simulink model "czwartasymulacja"  (R2024a)
settings: Solver=VariableStepAuto  StartTime=0.0  StopTime=150000  RelTol=1e-3
libraries: fl_lib x3, nesl_utility x3, BatteryCurrentManagement x1, batt_lib x1, BatteryEstimators x1
settings Model: Creator=jakub  LastModifiedBy=jakub

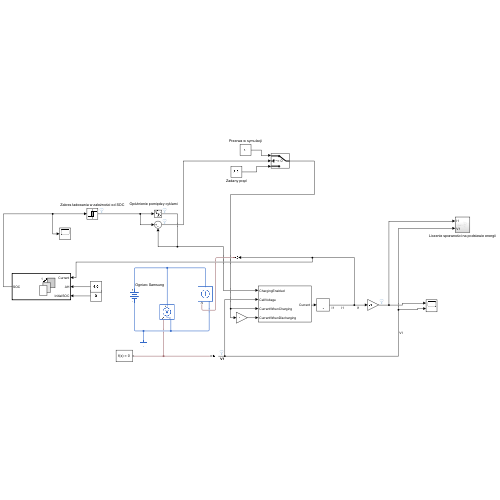
[thumbnail: Simulink's stored preview of the top-level diagram]
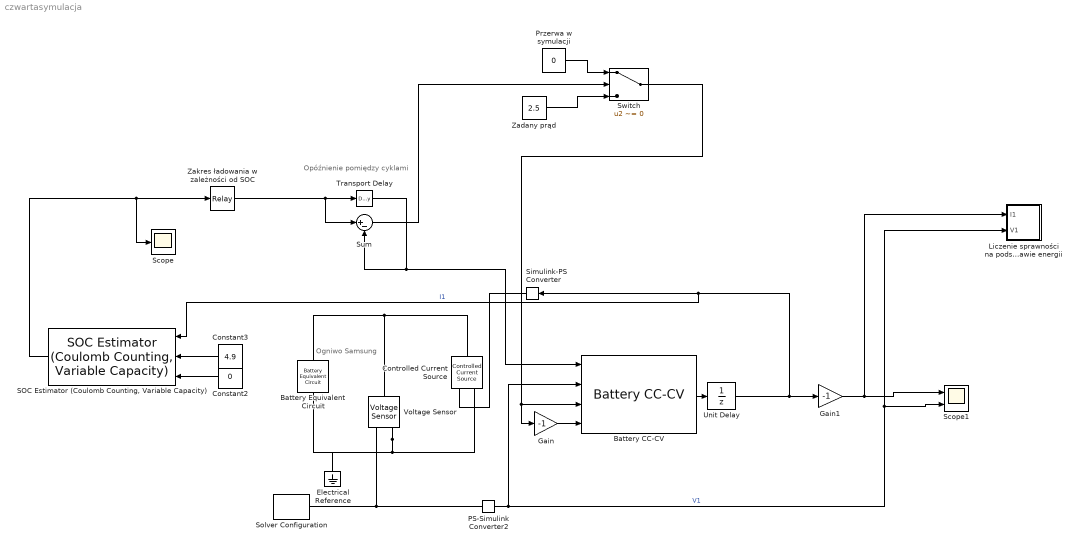
== system czwartasymulacja ==
  note: Ogniwo Samsung
  note: Opóźnienie pomiędzy cyklami
  Battery CC-CV : BatteryCurrentManagement/Battery CC-CV  MaxCellVoltage=4.28  Kp=1  Ki=5  Kaw=1  Kt=1  Ts=1
      settings: LibrarySourceBlock=batt_sl_lib/Current Management/Battery CC-CV
  Battery Equivalent Circuit : batt_lib/Cells/Battery Equivalent Circuit  BatteryCapacity=4900 mAh  ThermalModel=simscape.battery.enum.cells.BatteryThermalModel.ConstantTemperature  ExtrapolationMethod=simscape.enum.extrapolation.nearest  EnableFaultExotherm=false  TriggerTemperature=350 K  SOCBreakpoints=[0.01, 0.04, 0.06, 0.09, 0.11, 0.14, 0.16, 0.19, 0.21, 0.24, 0.26, 0.29, 0.31, 0.34, 0.36, 0.39, 0.41, 0.44, 0.46, 0.49, 0.51, 0.54, 0.56, 0.59, 0.61, 0.64, 0.66, 0.69, 0.71, 0.74, 0.76, 0.79, 0.81, 0.84, 0.86, 0.89]  TemperatureBreakpoints=[278, 293, 313] K  OpenCircuitVoltage=[3.5057, 3.566, 3.6337, 3.7127, 3.9259, 4.0777, 4.1928] V  OpenCircuitVoltageThermal=|  VoltageRange=[0, inf] V  HysteresisModel=simscape.battery.enum.cells.HysteresisModel.none  MaximumHysteresisVoltage=[0, 0, 0, 0, 0, 0, 0] V  InstantaneousHysteresisVoltage=[0, 0, 0, 0, 0, 0, 0] V  HysteresisRate=0.1  MaximumHysteresisVoltageThermal=[0, 0, 0; 0, 0, 0; 0, 0, 0; 0, 0, 0; 0, 0, 0; 0, 0, 0; 0, 0, 0] V  InstantaneousHysteresisVoltageThermal=[0, 0, 0; 0, 0, 0; 0, 0, 0; 0, 0, 0; 0, 0, 0; 0, 0, 0; 0, 0, 0] V  HysteresisRateThermal=0.1  ResistanceSOCBreakpoints=[.01, .1, .25, .5, .75, .9, 1]  ResistanceTemperatureBreakpoints=[278, 293, 313] K  CurrentDirectionality=simscape.battery.enum.cells.BatteryEnable.Disabled  R0=[.0085, .0085, .0087, .0082, .0083, .0085, .0085] Ohm  R0Thermal=|  DischargeR0=[.0085, .0085, .0087, .0082, .0083, .0085, .0085] Ohm  ChargeR0=[.0085, .0085, .0087, .0082, .0083, .0085, .0085] Ohm  ChargeR0Thermal=|  DischargeR0Thermal=|  SelfDischargeResistor=simscape.battery.enum.cells.BatteryEnable.Disabled  SelfDischargeR=7e3 Ohm  SelfDischargeRThermal=[8000, 7000, 6000] Ohm  RCPairs=simscape.battery.enum.cells.RCPairs.noDynamics  R1=[.0029, .0024, .0026, .0016, .0023, .0018, .0017] Ohm  Tau1=[36, 45, 105, 29, 77, 33, 39] s  R2=[.0029, .0024, .0026, .0016, .0023, .0018, .0017] Ohm  Tau2=[36, 45, 105, 29, 77, 33, 39] s  R3=[.0029, .0024, .0026, .0016, .0023, .0018, .0017] Ohm  Tau3=[36, 45, 105, 29, 77, 33, 39] s  DischargeR1=[.0029, .0024, .0026, .0016, .0023, .0018, .0017] Ohm  DischargeTau1=[36, 45, 105, 29, 77, 33, 39] s  ChargeR1=[.0029, .0024, .0026, .0016, .0023, .0018, .0017] Ohm  ChargeTau1=[36, 45, 105, 29, 77, 33, 39] s  DischargeR2=[.0029, .0024, .0026, .0016, .0023, .0018, .0017] Ohm  DischargeTau2=[36, 45, 105, 29, 77, 33, 39] s  ChargeR2=[.0029, .0024, .0026, .0016, .0023, .0018, .0017] Ohm  ChargeTau2=[36, 45, 105, 29, 77, 33, 39] s  DischargeR3=[.0029, .0024, .0026, .0016, .0023, .0018, .0017] Ohm  DischargeTau3=[36, 45, 105, 29, 77, 33, 39] s  ChargeR3=[.0029, .0024, .0026, .0016, .0023, .0018, .0017] Ohm  ChargeTau3=[36, 45, 105, 29, 77, 33, 39] s  R1Thermal=[.0109, .0029, .0013; .0069, .0024, .0012; .0047, .0026, .0013; .0034, .0016, .001; .0033, .0023, .0014; .0033, .0018, .0011; .0028, .0017, .0011] Ohm  Tau1Thermal=[20, 36, 39; 31, 45, 39; 109, 105, 61; 36, 29, 26; 59, 77, 67; 40, 33, 29; 25, 39, 33] s  R2Thermal=[.0109, .0029, .0013; .0069, .0024, .0012; .0047, .0026, .0013; .0034, .0016, .001; .0033, .0023, .0014; .0033, .0018, .0011; .0028, .0017, .0011] Ohm  Tau2Thermal=[20, 36, 39; 31, 45, 39; 109, 105, 61; 36, 29, 26; 59, 77, 67; 40, 33, 29; 25, 39, 33] s  R3Thermal=[.0109, .0029, .0013; .0069, .0024, .0012; .0047, .0026, .0013; .0034, .0016, .001; .0033, .0023, .0014; .0033, .0018, .0011; .0028, .0017, .0011] Ohm  Tau3Thermal=[20, 36, 39; 31, 45, 39; 109, 105, 61; 36, 29, 26; 59, 77, 67; 40, 33, 29; 25, 39, 33] s  DischargeR1Thermal=[.0109, .0029, .0013; .0069, .0024, .0012; .0047, .0026, .0013; .0034, .0016, .001; .0033, .0023, .0014; .0033, .0018, .0011; .0028, .0017, .0011] Ohm  DischargeTau1Thermal=[20, 36, 39; 31, 45, 39; 109, 105, 61; 36, 29, 26; 59, 77, 67; 40, 33, 29; 25, 39, 33] s  ChargeR1Thermal=[.0109, .0029, .0013; .0069, .0024, .0012; .0047, .0026, .0013; .0034, .0016, .001; .0033, .0023, .0014; .0033, .0018, .0011; .0028, .0017, .0011] Ohm  ChargeTau1Thermal=[20, 36, 39; 31, 45, 39; 109, 105, 61; 36, 29, 26; 59, 77, 67; 40, 33, 29; 25, 39, 33] s  DischargeR2Thermal=[.0109, .0029, .0013; .0069, .0024, .0012; .0047, .0026, .0013; .0034, .0016, .001; .0033, .0023, .0014; .0033, .0018, .0011; .0028, .0017, .0011] Ohm  DischargeTau2Thermal=[20, 36, 39; 31, 45, 39; 109, 105, 61; 36, 29, 26; 59, 77, 67; 40, 33, 29; 25, 39, 33] s  ChargeR2Thermal=[.0109, .0029, .0013; .0069, .0024, .0012; .0047, .0026, .0013; .0034, .0016, .001; .0033, .0023, .0014; .0033, .0018, .0011; .0028, .0017, .0011] Ohm  ChargeTau2Thermal=[20, 36, 39; 31, 45, 39; 109, 105, 61; 36, 29, 26; 59, 77, 67; 40, 33, 29; 25, 39, 33] s  DischargeR3Thermal=[.0109, .0029, .0013; .0069, .0024, .0012; .0047, .0026, .0013; .0034, .0016, .001; .0033, .0023, .0014; .0033, .0018, .0011; .0028, .0017, .0011] Ohm  DischargeTau3Thermal=[20, 36, 39; 31, 45, 39; 109, 105, 61; 36, 29, 26; 59, 77, 67; 40, 33, 29; 25, 39, 33] s  ChargeR3Thermal=[.0109, .0029, .0013; .0069, .0024, .0012; .0047, .0026, .0013; .0034, .0016, .001; .0033, .0023, .0014; .0033, .0018, .0011; .0028, .0017, .0011] Ohm  ChargeTau3Thermal=[20, 36, 39; 31, 45, 39; 109, 105, 61; 36, 29, 26; 59, 77, 67; 40, 33, 29; 25, 39, 33] s  CyclingAgingMethod=simscape.battery.enum.cells.CyclingAgingMethod.disabled  NumDisCycles=100  OCVChange=0  R0Change=0  CapacityChange=0  SelfDischargeRChange=0  R1Change=0  R2Change=0  R3Change=0  NumDisCyclesBreakpoints=[0, 100, 200, 300]  AgingTemperatureBreakpoints=[298.15, 323.15] K  OCVChangeVec=[0, 0, 0, 0]  R0ChangeVec=[0, 0, 0, 0]  CapacityChangeVec=[0, 0, 0, 0]  SelfDischargeRChangeVec=[0, 0, 0, 0]  R1ChangeVec=[0, 0, 0, 0]  R2ChangeVec=[0, 0, 0, 0]  R3ChangeVec=[0, 0, 0, 0]  OCVChangeThermal=[0, 0; 0, 0; 0, 0; 0, 0]  R0ChangeThermal=[0, 0; 0, 0; 0, 0; 0, 0]  CapacityChangeThermal=[0, 0; 0, 0; 0, 0; 0, 0]  SelfDischargeRChangeThermal=[0, 0; 0, 0; 0, 0; 0, 0]  R1ChangeThermal=[0, 0; 0, 0; 0, 0; 0, 0]  R2ChangeThermal=[0, 0; 0, 0; 0, 0; 0, 0]  R3ChangeThermal=[0, 0; 0, 0; 0, 0; 0, 0]  CalendarAgeResistance=simscape.battery.enum.cells.BatteryEnable.Disabled  CalendarAgeCapacity=simscape.battery.enum.cells.BatteryEnable.Disabled  CalendarAgingMethod=simscape.battery.enum.cells.CalendarAgingMethod.equation  StorageVariable=simscape.battery.enum.cells.StorageVariable.OCV  OCVDuringStorage=0.9  SOCDuringStorage=0.6  StorageTimeIntervals=[0] d  StorageTemperatures=[273] K  ResistanceScalingOCV=2.2134e6  ResistanceScalingOCVOffset=1.632e6  ResistanceExponentialIncrease=0.515833569 V  ResistanceTimeExponent=0.75  ResistanceAgeTemperatureBreakpoints=[273.15, 298.15, 323.15] K  ResistanceAgeTimeBreakpoints=[0, 90, 180, 270] d  PercentResistanceChange=[0, 0, 0]  ResistanceTimeBreakpoints=100 d  PercentResistanceChangeThermal=[0, 0, 0; 0, 0, 0; 0, 0, 0; 0, 0, 0]  CapacityScalingOCV=1.5097e07  CapacityScalingOCVOffset=8.3625e06  CapacityExponentialIncrease=0.6011 V  CapacityTimeExponent=0.75  CapacityAgeTemperatureBreakpoints=[273.15, 298.15, 323.15] K  CapacityAgeTimeBreakpoints=[0, 90, 180, 270] d  PercentCapacityChange=[0, 0, 0]  CapacityTimeBreakpoints=100 d  PercentCapacityChangeThermal=[0, 0, 0; 0, 0, 0; 0, 0, 0; 0, 0, 0]  SimulationTemperature=298.15 K  BatteryThermalMass=100 J/K  ReversibleHeatModel=simscape.battery.enum.cells.ReversibleHeatModel.Disabled  EntropicCoefficient=[0, 0, 0, 0, 0, 0, 0] mV/K  AddedResistance=1e5 Ohm  ShortedResistance=1e-6 Ohm  ExothermModel=simscape.battery.enum.cells.ExothermModel.analytical  TabulateWithSOC=false  SOCvecExotherm=[0, .5, 1]  CurrInterruptTempSOC=[420, 420, 420] K  TotalHeatOfReactionSOC=[23000, 23000, 23000] J  CurrentInterruptTemperature=420 K  TotalHeatOfReaction=23e3 J  ExothermOnsetTemperature=350 K  ExothermOnsetTempSOC=[350, 350, 350] K  OnsetTempRate=0.02 K/min  ActivationEnergy=160e3 J/mol  ActivationEnergySOC=[160000, 160000, 160000] J/mol  ReactionOrder=1  ReactionOrderSOC=[1, 1, 1]  TemperaturesFromARC=[323, 373, 423, 438, 463, 483, 513, 543, 545, 547, 549, 551, 553, 573, 623, 773, 923, 943, 1003, 1063, 1113, 1123, 1133, 1153, 1173] K  TemperatureRatesFromARC=[.0001, .001, .025, .2, .4, .6, 1.1, 1.3, 1.9, 3, 5, 11.6, 183.3, 191.6, 200, 208.3, 200, 175, 8.33, 1.33, .33, .2, .13, .0017, .00017] K/s  TempRateVecARCSOC=repmat([.0001, .001, .025, .2, .4, .6, 1.1, 1.3, 1.9, 3, 5, 11.6, 183.3, 191.6, 200, 208.3, 200, 175, 8.33, 1.33, .33, .2, .13, .0017, .00017]', 1, 3) K/s  PercentThermalMassVented=40  PercentThermalMassVentedSOC=[40, 40, 40]  EnableFaultAddRes=false  EnableFaultShort=false  faultTriggerType=simscape.fault.triggertype.external  stateOfCharge_specify=on  stateOfCharge_priority=High  stateOfCharge=0  stateOfCharge_nominal_specify=off  stateOfCharge_nominal_value=1  stateOfCharge_nominal_unit=1  numCycles_specify=off  numCycles_priority=High  numCycles=0.1  numCycles_nominal_specify=off  numCycles_nominal_value=1  numCycles_nominal_unit=1  batteryVoltage_specify=off  batteryVoltage_priority=None  batteryVoltage=0 V  batteryVoltage_nominal_specify=off  batteryVoltage_nominal_value=1  batteryVoltage_nominal_unit=V  batteryCurrent_specify=off  batteryCurrent_priority=None  batteryCurrent=0 A  batteryCurrent_nominal_specify=off  batteryCurrent_nominal_value=1  batteryCurrent_nominal_unit=A  batteryTemperature_specify=off  batteryTemperature_priority=High  batteryTemperature=298.15 K  batteryTemperature_nominal_specify=off  batteryTemperature_nominal_value=1  batteryTemperature_nominal_unit=K  hysteresisState_specify=off  hysteresisState_priority=High  hysteresisState=0  hysteresisState_nominal_specify=off  hysteresisState_nominal_value=1  hysteresisState_nominal_unit=1  isExothermFaulted_specify=off  isExothermFaulted_priority=None  isExothermFaulted=0  isExothermFaulted_nominal_specify=off  isExothermFaulted_nominal_value=1  isExothermFaulted_nominal_unit=1  isCurrentInterruptionTempExceeded_specify=off  isCurrentInterruptionTempExceeded_priority=None  isCurrentInterruptionTempExceeded=0  isCurrentInterruptionTempExceeded_nominal_specify=off  isCurrentInterruptionTempExceeded_nominal_value=1  isCurrentInterruptionTempExceeded_nominal_unit=1  reactionHeatRate_specify=off  reactionHeatRate_priority=None  reactionHeatRate=0 W  reactionHeatRate_nominal_specify=off  reactionHeatRate_nominal_value=1  reactionHeatRate_nominal_unit=W  reactionExtent_specify=off  reactionExtent_priority=None  reactionExtent=0  reactionExtent_nominal_specify=off  reactionExtent_nominal_value=1  reactionExtent_nominal_unit=1
      OpenCircuitVoltageThermal=|
      | [
      |        2.60, 2.58, 2.55;
      |        2.78, 2.76, 2.73;
      |        2.96, 2.94, 2.91;
      |        3.14, 3.11, 3.09;
      |        3.27, 3.24, 3.22;
      |        3.31, 3.28, 3.26;
      |        3.35, 3.33, 3.30;
      |        3.39, 3.37, 3.34;
      |        3.42, 3.40, 3.37;
      |        3.44, 3.42, 3.39;
      |        3.46, 3.44, 3.41;
      |        3.49, 3.47, 3.44;
      |        3.51, 3.49, 3.46;
      |        3.54, 3.52, 3.48;
      |        3.56, 3.54, 3.51;
      |        3.58, 3.56, 3.53;
      |        3.61, 3.59, 3.56;
      |        3.64, 3.62, 3.58;
      |        3.66, 3.64, 3.61;
      |        3.69, 3.67, 3.63;
      |        3.71, 3.69, 3.66;
      |        3.73, 3.71, 3.69;
      |        3.76, 3.74, 3.71;
      |        3.79, 3.77, 3.73;
      |        3.81, 3.79, 3.76;
      |        3.83, 3.81, 3.79;
      |        3.86, 3.84, 3.81;
      |        3.88, 3.86, 3.83;
      |        3.91, 3.89, 3.86;
      |        3.94, 3.92, 3.89;
      |        3.97, 3.95, 3.92;
      |        3.99, 3.97, 3.94;
      |        4.02, 4.00, 3.97;
      |        4.04, 4.03, 4.00;
      |        4.07, 4.05, 4.02;
      |        4.19, 4.19, 4.19
      | ] V
      R0Thermal=|
      | [0.0117, 0.0085, 0.009;
      |  0.011,  0.0085, 0.009;
      |  0.0114, 0.0087, 0.0092;
      |  0.0107, 0.0082, 0.0088;
      |  0.0107, 0.0083, 0.0091;
      |  0.0113, 0.0085, 0.0089;
      |  0.0116, 0.0085, 0.0089]
      |  Ohm
      ChargeR0Thermal=|
      | [0.0499, 0.0363, 0.0384, 0.0470, 0.0363, 0.0384, 0.0487, 0.0371, 0.0393, 0.0457, 0.0350, 0.0376, 0.0457, 0.0354, 0.0388, 0.0482, 0.0363, 0.0380, 0.0495, 0.0363, 0.0380]
      |  Ohm
      DischargeR0Thermal=|
      | [0.0499, 0.0363, 0.0384, 0.0470, 0.0363, 0.0384, 0.0487, 0.0371, 0.0393, 0.0457, 0.0350, 0.0376, 0.0457, 0.0354, 0.0388, 0.0482, 0.0363, 0.0380, 0.0495, 0.0363, 0.0380]
      |  Ohm
      settings: InternalSimscapePortConfiguration="{\"Bottom\":[],\"Left\":[{\"id\":\"p\",\"label\":\"+\",\"type\":\"foundation.electrical.electrical\"}],\"Right\":[{\"id\":\"n\",\"label\":\"-\",\"type\":\"foundation.electrical.electrical\"}],\"Top\":[]}"
  Constant2 : Constant  Value=0
  Constant3 : Constant  Value=4.9
  Controlled Current Source : fl_lib/Electrical/Electrical Sources/Controlled Current Source
  Electrical Reference : fl_lib/Electrical/Electrical Elements/Electrical Reference
  Gain : Gain  Gain=-1
  Gain1 : Gain  Gain=-1
  Liczenie sprawności na podstawie energii : Subsystem
  PS-Simulink Converter2 : nesl_utility/PS-Simulink Converter  PhysicalDomain=network_engine_domain  SubClassName=ps_output  LeftPortType=input  RightPortType=output  PseudoPeriodic=off  Frequencies=[]  VectorFormat=inherit  Unit=inherit  AffineConversion=off
  Przerwa w symulacji : Constant  Value=0
  "SOC Estimator (Coulomb Counting, Variable Capacity)" : BatteryEstimators/SOC Estimator (Coulomb Counting, Variable Capacity)  CurrentInputPartition=on  Ts=1
      settings: LibrarySourceBlock=|
      | batt_sl_lib/Estimators/SOC Estimator
      | (Coulomb Counting, Variable Capacity)
  Scope : Scope
  Scope1 : Scope  NumInputPorts=2
  Simulink-PS Converter : nesl_utility/Simulink-PS Converter  PhysicalDomain=network_engine_domain  SubClassName=ps_input  LeftPortType=input  RightPortType=output  PseudoPeriodic=off  Frequencies=[]  NoiseDistribution=none  NoiseParameters=[]  Unit=1  AffineConversion=off  FilteringAndDerivatives=provide  SimscapeFilterOrder=1  InputFilterTimeConstant=0.001  UdotUserProvided=0
  Solver Configuration : nesl_utility/Solver Configuration  PhysicalDomain=network_engine_domain  SubClassName=solver  LeftPortType=input  RightPortType=generic  Tones=[]  Harmonics=[]  SimulateNoise=off  Profile=off  UseLocalSampling=off  EnableSwitchedLinearOptims=on  FrequencyDomain=off  UseCCode=off  RelTol=0.001  AbsTol=0.001  MinStep=1e-09  ToWorkspace=off  RevertToSquareIcSolve=off  NumHomotopyIterations=100  PhasorMode=off  PhasorModeNumHarmonics=1  ConsistencySolver=NEWTON_XTOL_AFTER_FTOL  IndexReductionMethod=DerivativeReplacement  DoDC=off  ResidualTolerance=1e-09  ConsistencyTolSource=GLOBAL  ConsistencyAbsTol=0.001  ConsistencyRelTol=0.001  ConsistencyTolFactor=0.001  UseLocalSolver=off  LocalSolverChoice=NE_BACKWARD_EULER_ADVANCER  ResolveIndetEquations=on  FunctionEvalNumThread=1  LocalSolverSampleTime=0.001  DoFixedCost=off  MaxNonlinIter=3  MaxModeIter=2  ComputeImpulses=off  ImpulseIterations=2  LinearAlgebra=auto  LinearAlgebraNumThread=0  EquationFormulation=NE_TIME_EF  DelaysMemoryBudget=1024  AutomaticFiltering=on  FilteringTimeConstant=0.001  PartitionStorageMethod=AS_NEEDED  PartitionMemoryBudget=1024  PartitionMethod=ROBUST  MultibodyUseLocalSolver=off  MultibodyLocalSolverChoice=ODE1  MultibodyLocalSolverSampleTime=0.001
  Sum : Sum  Inputs=|+-
  Switch : Switch  Criteria=u2 ~= 0  SaturateOnIntegerOverflow=off  InputSameDT=off
  Transport Delay : TransportDelay  DelayTime=5000
  Unit Delay : UnitDelay  SampleTime=-1  HasFrameUpgradeWarning=on
  Voltage Sensor : fl_lib/Electrical/Electrical Sensors/Voltage Sensor
  Zadany prąd : Constant  Value=2.5
  Zakres ładowania w zależności od SOC : Relay  OnSwitchValue=0.98  OffSwitchValue=0.01  OnOutputValue=0  OffOutputValue=1
  wires:
  Gain/1 -> Battery CC-CV/4
  Battery CC-CV/1 -> Unit Delay/1
  Unit Delay/1 -> "SOC Estimator (Coulomb Counting, Variable Capacity)"/1, Simulink-PS Converter/1, Gain1/1  "I1"
  Zakres ładowania w zależności od SOC/1 -> Sum/1, Transport Delay/1
  Transport Delay/1 -> Sum/2, Battery CC-CV/1
  Sum/1 -> Switch/2
  Switch/1 -> Gain/1, Battery CC-CV/3
  Przerwa w symulacji/1 -> Switch/1
  PS-Simulink Converter2/1 -> Liczenie sprawności na podstawie energii/2(V1), Scope1/2, Battery CC-CV/2  "V1"
  Zadany prąd/1 -> Switch/3
  "SOC Estimator (Coulomb Counting, Variable Capacity)"/1 -> Scope/1, Zakres ładowania w zależności od SOC/1
  Constant3/1 -> "SOC Estimator (Coulomb Counting, Variable Capacity)"/2
  Constant2/1 -> "SOC Estimator (Coulomb Counting, Variable Capacity)"/3
  Gain1/1 -> Liczenie sprawności na podstawie energii/1(I1), Scope1/1
  connections:
  Controlled Current Source/RConn1 -- Simulink-PS Converter/RConn1
  Controlled Current Source/LConn1 -- Battery Equivalent Circuit/LConn1 -- Voltage Sensor/LConn1
  Voltage Sensor/RConn2 -- Controlled Current Source/RConn2 -- Battery Equivalent Circuit/RConn1 -- Electrical Reference/LConn1
  Voltage Sensor/RConn1 -- Solver Configuration/RConn1 -- PS-Simulink Converter2/LConn1

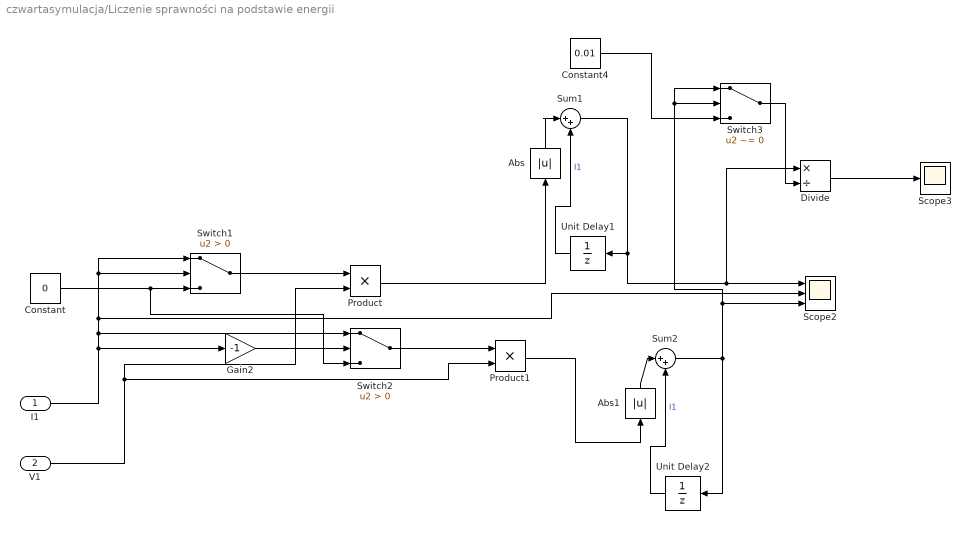
== system czwartasymulacja/Liczenie sprawności na podstawie energii ==
  I1 : Inport
  V1 : Inport  Port=2
  Abs : Abs  SaturateOnIntegerOverflow=off
  Abs1 : Abs  SaturateOnIntegerOverflow=off
  Constant : Constant  Value=0
  Constant4 : Constant  Value=0.01
  Divide : Product  Inputs=*/
  Gain2 : Gain  Gain=-1
  Product : Product
  Product1 : Product
  Scope2 : Scope  NumInputPorts=3
  Scope3 : Scope
  Sum1 : Sum  Inputs=|++
  Sum2 : Sum  Inputs=|++
  Switch1 : Switch  Criteria=u2 > Threshold  SaturateOnIntegerOverflow=off  InputSameDT=off
  Switch2 : Switch  Criteria=u2 > Threshold  SaturateOnIntegerOverflow=off  InputSameDT=off
  Switch3 : Switch  Criteria=u2 ~= 0  SaturateOnIntegerOverflow=off  InputSameDT=off
  Unit Delay1 : UnitDelay  HasFrameUpgradeWarning=on
  Unit Delay2 : UnitDelay  HasFrameUpgradeWarning=on
  wires:
  Abs1/1 -> Sum2/1
  V1/1 -> Product1/2, Product/2
  I1/1 -> Switch2/1, Scope2/2, Switch1/1, Switch1/2, Gain2/1
  Sum1/1 -> Divide/1, Scope2/1, Unit Delay1/1
  Constant/1 -> Switch2/3, Switch1/3
  Switch3/1 -> Divide/2
  Sum2/1 -> Switch3/1, Switch3/2, Scope2/3, Unit Delay2/1
  Unit Delay2/1 -> Sum2/2  "I1"
  Switch1/1 -> Product/1
  Unit Delay1/1 -> Sum1/2  "I1"
  Product/1 -> Abs/1
  Divide/1 -> Scope3/1
  Product1/1 -> Abs1/1
  Constant4/1 -> Switch3/3
  Switch2/1 -> Product1/1
  Abs/1 -> Sum1/1
  Gain2/1 -> Switch2/2
